simulink model "oddparityfourbitgenerator"  (R2021b)
settings: Solver=VariableStepAuto  StartTime=0.0  StopTime=1  RelTol=1e-3
settings Model: Creator=Joshua  LastModifiedBy=Joshua

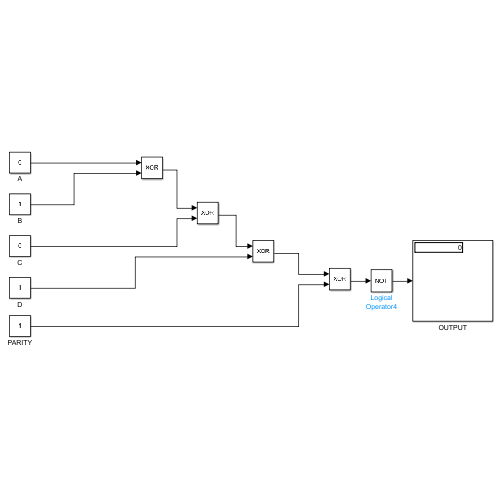
[thumbnail: Simulink's stored preview of the top-level diagram]
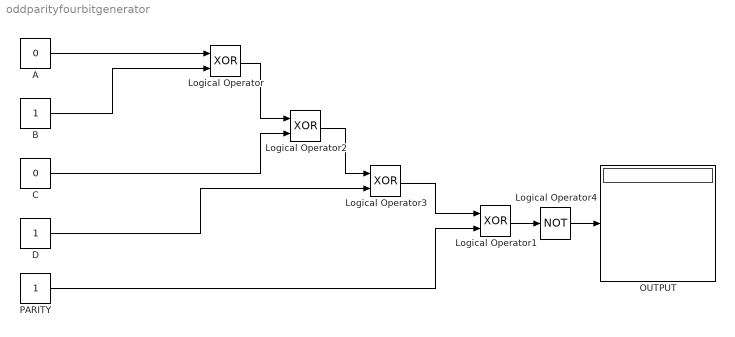
== system oddparityfourbitgenerator ==
  A : Constant  Value=0
  B : Constant
  C : Constant  Value=0
  D : Constant
  Logical Operator{,1..3} (4 alike) : Logic  Operator=XOR  AllPortsSameDT=off  OutDataTypeStr=boolean
  Logical Operator4 : Logic  Operator=NOT  AllPortsSameDT=off  OutDataTypeStr=boolean
  OUTPUT : Display
  PARITY : Constant
  wires:
  D/1 -> Logical Operator3/2
  Logical Operator3/1 -> Logical Operator1/1
  C/1 -> Logical Operator2/2
  PARITY/1 -> Logical Operator1/2
  A/1 -> Logical Operator/1
  Logical Operator/1 -> Logical Operator2/1
  Logical Operator2/1 -> Logical Operator3/1
  B/1 -> Logical Operator/2
  Logical Operator1/1 -> Logical Operator4/1
  Logical Operator4/1 -> OUTPUT/1
